simulink model "VDSE_2019a"  (R2019a)
settings: Solver=ode5  StartTime=0.0  StopTime=T_simulation  FixedStep=simulation_step_time  RelTol=1e-3
values from neighbouring files (symbols this model uses):
  A = 2    [vehicle_parameters_script.m]
  bump_height = 0    [vehicle_parameters_script.m]
  bump_length = 1    [vehicle_parameters_script.m]
  bump_time = 1    [vehicle_parameters_script.m]
  Bxf = 17.156    [BCD_Parameters.m]
  Bxr = 17.156    [BCD_Parameters.m]
  Byf = 12.71    [BCD_Parameters.m]
  Byr = 12.71    [BCD_Parameters.m]
  cd = 0.35    [vehicle_parameters_script.m]
  central_diff = 1    [vehicle_parameters_script.m]
  cF = 5000    [vehicle_parameters_script.m]
  clF = -0.15    [vehicle_parameters_script.m]
  clR = -0.20    (= -0.2)    [vehicle_parameters_script.m]
  cp_FA = 30    [vehicle_parameters_script.m]
  cp_RA = 13    [vehicle_parameters_script.m]
  cR = 5000    [vehicle_parameters_script.m]
  ctF = tireF.VERTICAL_DAMPING    [vehicle_parameters_script.m]
  ctR = tireR.VERTICAL_DAMPING    [vehicle_parameters_script.m]
  Cxf = 1.406    [BCD_Parameters.m]
  Cxr = 1.406    [BCD_Parameters.m]
  Cyf = 1.63    [BCD_Parameters.m]
  Cyr = 1.63    [BCD_Parameters.m]
  Dxf = 1.2    [BCD_Parameters.m]
  Dxr = 1.2    [BCD_Parameters.m]
  Dyf = 1.1    [BCD_Parameters.m]
  Dyr = 1.8    [BCD_Parameters.m]
  enableDriverControl = 0    [vehicle_parameters_script.m]
  enableLongDynamics = 1    [vehicle_parameters_script.m]
  enablePowertrain = 1    [vehicle_parameters_script.m]
  front_dr = 3.8    [vehicle_parameters_script.m]
  g = 9.806    [vehicle_parameters_script.m]
  Gear_numbers = [1 2 3 4 5 6]    [vehicle_parameters_script.m]
  GR = [2.9 1.8 1.3 1 0.85 0.75]    [vehicle_parameters_script.m]
  hcog = 0.5    [vehicle_parameters_script.m]
  hpc = 0.0    (= 0)    [vehicle_parameters_script.m]
  hrcF = 0.3    [vehicle_parameters_script.m]
  hrcg = (hrcF*lR+hrcR*lF)/(lF+lR)    (= 0.25108)    [vehicle_parameters_script.m]
  hrcR = 0.2    [vehicle_parameters_script.m]
  huFcog = 0.32    [vehicle_parameters_script.m]
  huRcog = 0.32    [vehicle_parameters_script.m]
  initial_gear = 1    [vehicle_parameters_script.m]
  JwF = 2.45    [vehicle_parameters_script.m]
  JwR = 2.45    [vehicle_parameters_script.m]
  Jx = 430    [vehicle_parameters_script.m]
  Jy = 1309    [vehicle_parameters_script.m]
  Jz = 1461    [vehicle_parameters_script.m]
  kF = 40000    [vehicle_parameters_script.m]
  kR = 35000    [vehicle_parameters_script.m]
  kRF = 0    [vehicle_parameters_script.m]
  kRR = 0    [vehicle_parameters_script.m]
  ktF = tireF.VERTICAL_STIFFNESS    [vehicle_parameters_script.m]
  ktR = tireR.VERTICAL_STIFFNESS    [vehicle_parameters_script.m]
  lF = 1.223    [vehicle_parameters_script.m]
  lR = l-lF    (= 1.277)    [vehicle_parameters_script.m]
  m = 1310    [vehicle_parameters_script.m]
  max_pressure = 1000    [vehicle_parameters_script.m]
  maxrpm = 4000    [vehicle_parameters_script.m]
  mF = 45    [vehicle_parameters_script.m]
  minrpm = 1500    [vehicle_parameters_script.m]
  mR = 50    [vehicle_parameters_script.m]
  output_samping_time = 0.001    [vehicle_parameters_script.m]
  phi0 = 0    [vehicle_parameters_script.m]
  phi_dot0 = 0    [vehicle_parameters_script.m]
  psi0 = 0    [vehicle_parameters_script.m]
  psi_dot0 = 0    [vehicle_parameters_script.m]
  rear_dr = 3.8    [vehicle_parameters_script.m]
  requested_speed = 100/3.6    (= 27.7777777778)    [vehicle_parameters_script.m]
  rF = tireF.UNLOADED_RADIUS    [vehicle_parameters_script.m]
  rho = 1.2    [vehicle_parameters_script.m]
  RPMME = Engine(:,1)    [vehicle_parameters_script.m]
  rR = tireR.UNLOADED_RADIUS    [vehicle_parameters_script.m]
  steer_ratio = 13.25    [vehicle_parameters_script.m]
  TFL = 0    [vehicle_parameters_script.m]
  TFR = 0    [vehicle_parameters_script.m]
  theta0 = 0    [vehicle_parameters_script.m]
  theta_dot0 = 0    [vehicle_parameters_script.m]
  TorqueME = []    [vehicle_parameters_script.m]
  TRL = 0    [vehicle_parameters_script.m]
  TRR = 0    [vehicle_parameters_script.m]
  Vx0 = 100/3.6    (= 27.7777777778)    [vehicle_parameters_script.m]
  Vy0 = 0    [vehicle_parameters_script.m]
  Vz0 = 0    [vehicle_parameters_script.m]
  wF = 1.578    [vehicle_parameters_script.m]
  wR = 1.544    [vehicle_parameters_script.m]
  x0 = 0    [vehicle_parameters_script.m]
  xcog_overall = (2*mR*xR+2*xF*mF+m*xs)/(m+2*mF+2*mR)    (= 1.23475333333)    [vehicle_parameters_script.m]
  y0 = 0    [vehicle_parameters_script.m]
  z0 = 0    [vehicle_parameters_script.m]
  zFL0 = 0    [vehicle_parameters_script.m]
  zFL_dot0 = 0    [vehicle_parameters_script.m]
  zFR0 = 0    [vehicle_parameters_script.m]
  zFR_dot0 = 0    [vehicle_parameters_script.m]
  zRL0 = 0    [vehicle_parameters_script.m]
  zRL_dot0 = 0    [vehicle_parameters_script.m]
  zRR0 = 0    [vehicle_parameters_script.m]
  zRR_dot0 = 0    [vehicle_parameters_script.m]
undefined symbols (not defined in the file or in its folder): exf, exr, eyf, eyr, FNOMINf, FNOMINr, PCX1f, PCX1r, PCY1f, PCY1r, PDX1f, PDX1r, PDX2f, PDX2r, PDY1f, PDY1r, PDY2f, PDY2r, PDY3f, PDY3r, PEX1f, PEX1r, PEX2f, PEX2r, PEX3f, PEX3r, PEX4f, PEX4r, PEY1f, PEY1r, PEY2f, PEY2r, PEY3f, PEY3r, PEY4f, PEY4r, PHX1f, PHX1r, PHX2f, PHX2r, PHY1f, PHY1r, PHY2f, PHY2r, PHY3f, PHY3r, PKX1f, PKX1r, PKX2f, PKX2r, PKX3f, PKX3r, PKY1f, PKY1r, PKY2f, PKY2r, PKY3f, PKY3r, PVX1f, PVX1r ... (+122)
libraries: simulink x7, mfeval_LIB x4
(part 5 of 6)

== matlab function VDSE_2019a/14-DOF VEHICLE MODEL/WHEEL ASSEMBLY/WHEEL ASSEMBLY MFEVAL/TIRE VELOCITIES ==
  data: deltaFL input; VFLx output; VFLy output; VFRx output; VFRy output; VRLx output; VRLy output; VRRx output; deltaFR input; deltaRL input; deltaRR input; V input; beta input; psidot input; VRRy output; lF input; lR input; wFL input; wFR input; wRL input; wRR input
function [VFLx, VFLy, VFRx, VFRy, VRLx, VRLy, VRRx, VRRy] = ConversiontoCorners(deltaFL,deltaFR,deltaRL,deltaRR,...
    V, beta, psidot,  lF, lR, wFL, wFR, wRL, wRR)
% Geometric calcs
lFL = sqrt(lF^2+wFL^2); gammaFL = atan2(wFL,lF);
lFR = sqrt(lF^2+wFR^2); gammaFR = atan2(wFR,lF);
lRL = sqrt(lR^2+wRL^2); gammaRL = atan2(wRL,lR);
lRR = sqrt(lR^2+wRR^2); gammaRR = atan2(wRR,lR);

VFLx = V*cos(deltaFL - beta) - psidot*lFL*sin(gammaFL - deltaFL);
VFLy = - V*sin(deltaFL - beta) + psidot*lFL*cos(gammaFL - deltaFL);
VFRx = V*cos(deltaFR - beta) + psidot*lFR*sin(gammaFR + deltaFR);
VFRy = - V*sin(deltaFR - beta) + psidot*lFR*cos(gammaFR + deltaFR);
VRLx = V*cos(deltaRL - beta) - psidot*lRL*sin(gammaRL + deltaRL);
VRLy = -V*sin(deltaRL - beta) - psidot*lRL*cos(gammaRL + deltaRL);
VRRx = V*cos(deltaRR - beta) + psidot*lRR*sin(gammaRR - deltaRR);
VRRy = -V*sin(deltaRR - beta) - psidot*lRR*cos(gammaRR - deltaRR);

end

== matlab function VDSE_2019a/14-DOF VEHICLE MODEL/WHEEL ASSEMBLY/WHEEL ASSEMBLY MFEVAL/WHEEL DYNAMICS ==
  data: rF input; rR input; JwF input; JwR input; omega_dot output size=[1 4]; fFLx input; fFRx input; fRLx input; fRRx input; TFL input; TFR input; TRL input; TRR input
function omega_dot  = TIRES(rF, rR, JwF, JwR, fFLx, fFRx, fRLx, fRRx,TFL,TFR,TRL,TRR)

%Wheel Dynamics
domegaFL = (TFL - fFLx*rF)/(JwF);
domegaFR = (TFR - fFRx*rF)/(JwF);
domegaRL = (TRL - fRLx*rR)/(JwR);
domegaRR = (TRR - fRRx*rR)/(JwR);

omega_dot = [domegaFL, domegaFR, domegaRL, domegaRR];

end

== matlab function VDSE_2019a/14-DOF VEHICLE MODEL/SUSPENSION/REAR SUSPENSION/SUSPENSION RL/RL/MATLAB Function ==
  data: mR input; wR input; lR input; cR input; kR input; kRR input; ctR input; ktR input; g input; yRL_road input; yRL_road_dot input; zRL_dot_dot output; z input; Vz input; phi input; phi_dot input; theta input; theta_dot input; zRR input; zRL input; zRL_dot input
function zRL_dot_dot = zRL(mR,wR,lR,cR,kR,kRR,ctR,ktR,g,yRL_road,yRL_road_dot,z,Vz,phi,phi_dot,theta,theta_dot,zRR,zRL,zRL_dot)
% Parameters:
% mR = half rear unsprung mass [kg]
% cR = rear damping damping rate [Ns/m]
% kR = rear spring stiffness [N/m]
% kRR = rear antiroll bar stiffness [N/m]
% wR = rear trackwidth [m]
% g = gravitational acceleration [m/s^2]
%
% Annotations:
% z = sprung mass vertical displacement [m]
% Vz = sprung mass vertical velocity [m/s]
% zij = unsprung vertical displacement [m]
% zij_dot = unsprung vertical velocity [m/s]
% zij_dot_dot = unsprung vertical acceleration [m/s^2]
% theta = pitch angle [rad]
% theta_dot = pitch angular velocity [rad/s]
% phi = roll angle [rad]
% phi_dot  = roll angular velocity [rad/s]
% y_rear_road = rear axle's road input displacement [m]
% y_rear_road_dot = rear axle's road input velocity [m/s]
%
% i: F, R = Front, Rear
% j: R, L = Right, Left

% Summation of forces:
sum = -cR*(Vz-zRL_dot+wR/2*phi_dot+lR*theta_dot) - kR*(z-zRL+wR/2*phi+lR*theta) - kRR/wR*(phi-(zRL-zRR)/wR) ...
    +ktR*(zRL-yRL_road)+ctR*(zRL_dot-yRL_road_dot)+mR*g;

% Calculation of RR unsprung mass vertical acceleration:
zRL_dot_dot = -sum/mR;

end

== matlab function VDSE_2019a/14-DOF VEHICLE MODEL/SUSPENSION/REAR SUSPENSION/SUSPENSION RR/RR/MATLAB Function ==
  data: mR input; wR input; lR input; cR input; kR input; kRR input; ctR input; ktR input; g input; yRR_road input; yRR_road_dot input; zRR_dot_dot output; z input; Vz input; phi input; phi_dot input; theta input; theta_dot input; zRL input; zRR input; zRR_dot input
function zRR_dot_dot = zRR(mR,wR,lR,cR,kR,kRR,ctR,ktR,g,yRR_road,yRR_road_dot,z,Vz,phi,phi_dot,theta,theta_dot,zRL,zRR,zRR_dot)
% Parameters:
% mR = half rear unsprung mass [kg]
% cR = rear damping damping rate [Ns/m]
% kR = rear spring stiffness [N/m]
% kRR = rear antiroll bar stiffness [N/m]
% wR = rear trackwidth [m]
% g = gravitational acceleration [m/s^2]
%
% Annotations:
% z = sprung mass vertical displacement [m]
% Vz = sprung mass vertical velocity [m/s]
% zij = unsprung vertical displacement [m]
% zij_dot = unsprung vertical velocity [m/s]
% zij_dot_dot = unsprung vertical acceleration [m/s^2]
% theta = pitch angle [rad]
% theta_dot = pitch angular velocity [rad/s]
% phi = roll angle [rad]
% phi_dot  = roll angular velocity [rad/s]
% y_rear_road = rear axle's road input displacement [m]
% y_rear_road_dot = rear axle's road input velocity [m/s]
%
% i: F, R = Front, Rear
% j: R, L = Right, Left

% Summation of forces:
sum = -cR*(Vz-zRR_dot-wR/2*phi_dot+lR*theta_dot) - kR*(z-zRR-wR/2*phi+lR*theta)...
    +kRR/wR*(phi - (zRL-zRR)/wR)+ktR*(zRR-yRR_road)+ ctR*(zRR_dot-yRR_road_dot) + mR*g;
% Calculation of RR unsprung mass vertical acceleration:
zRR_dot_dot = -sum/mR; 

end

== matlab function VDSE_2019a/14-DOF VEHICLE MODEL/EQUATIONS OF MOTION FOR CHASSIS/Vertical Dynamics/VERTICAL DYNAMICS ==
  data: m input; g input; lF input; Vz_dot output; lR input; wF input; wR input; kF input; kR input; cF input; cR input; phi input; phi_dot input; theta input; theta_dot input; zFL input; zFL_dot input; zFR input; zFR_dot input; zRL input; zRL_dot input; zRR input; zRR_dot input; Vx input; Vy input; fFLz_aero input; fFRz_aero input; fRLz_aero input; fRRz_aero input; z input; z_dot input
function Vz_dot = vertical_dynamics(m,g,lF,lR,wF,wR,kF,kR,cF,cR,phi,phi_dot,...
    theta,theta_dot,zFL,zFL_dot,zFR,zFR_dot,zRL,zRL_dot,zRR,zRR_dot,Vx,Vy,...
    fFLz_aero, fFRz_aero, fRLz_aero, fRRz_aero,z,z_dot)
% Parameters:
% m = sprung mass [kg]
% cF = front damping damping rate [Ns/m]
% cR = rear damping damping rate [Ns/m]
% kF = front spring stiffness [N/m]
% kR = rear spring stiffness [N/m]
% lF = front wheel base [m]
% lR = rear wheel base [m]
% wF = front trackwidth [m]
% wR = rear trackwidth [m]
% g = gravitational acceleration [m/s^2]
%
% Annotations:
% z = sprung mass vertical displacement [m]
% Vz = sprung mass vertical velocity [m/s]
% Vz_dot = sprung mass vertical acceleration [m/s^2]
% zij = unsprung vertical displacement [m]
% zij_dot = unsprung vertical velocity [m/s]
% fijz_aero = downforces applied on the chassis [N]
% theta = pitch angle [rad]
% theta_dot = pitch angular velocity [rad/s]
% phi = roll angle [rad]
% phi_dot  = roll angular velocity [rad/s]
% Vy = vehicle's lateral velocity [m/s]
% Vx = vehicle's longitudinal velocity [m/s]
%
% i: F, R = Front, Rear
% j: R, L = Right, Left

% Summation of forces:
sum=cF*(z_dot-zFL_dot+(wF/2)*phi_dot-lF*theta_dot)...
    +cF*(z_dot-zFR_dot-(wF/2)*phi_dot-lF*theta_dot)...
    +cR*(z_dot-zRL_dot+(wR/2)*phi_dot+lR*theta_dot)...
    +cR*(z_dot-zRR_dot-(wR/2)*phi_dot+lR*theta_dot)...
    +kF*(z-zFL+(wF/2)*phi-lF*theta)...
    +kF*(z-zFR-(wF/2)*phi-lF*theta)...
    +kR*(z-zRL+(wR/2)*phi+lR*theta)...
    +kR*(z-zRR-(wR/2)*phi+lR*theta)...
    +m*g+m*Vx*theta_dot-m*Vy*phi_dot...
    +fFLz_aero+fFRz_aero+fRLz_aero+fRRz_aero;

% Calculation of vertical acceleration of sprung mass (including tangential terms):
Vz_dot=-sum/m;
end

== matlab function VDSE_2019a/14-DOF VEHICLE MODEL/EQUATIONS OF MOTION FOR CHASSIS/Roll Dynamics/ROLL DYNAMICS ==
  data: Jx input; g input; lF input; phi_dot_dot output; lR input; wF input; wR input; kF input; kR input; kRF input; kRR input; cF input; cR input; z input; z_dot input; theta input; theta_dot input; zFL input; zFL_dot input; zFR input; zFR_dot input; zRL input; zRL_dot input; zRR input; zRR_dot input; ay input; hrcg input; hcog input; m input; fFLz_aero input; fFRz_aero input; fRLz_aero input; fRRz_aero input; phi input; phi_dot input
function phi_dot_dot = roll_dynamics(Jx,g,lF,lR,wF,wR,kF,kR,kRF,kRR,cF,cR,z,z_dot,theta,theta_dot,...
    zFL,zFL_dot,zFR,zFR_dot,zRL,zRL_dot,zRR,zRR_dot,ay,hrcg,hcog,m,...
    fFLz_aero,fFRz_aero,fRLz_aero,fRRz_aero,phi,phi_dot)

% Parameters:
% m = sprung mass [kg]
% Jx = roll moment of inertial [kgm^2]
% cF = front damping damping rate [Ns/m]
% cR = rear damping damping rate [Ns/m]
% kF = front spring stiffness [N/m]
% kR = rear spring stiffness [N/m]
% kRF = front antiroll bar stiffness [N/m]
% kRR = front antiroll bar stiffness [N/m]
% lF = front wheel base [m]
% lR = rear wheel base [m]
% wF = front trackwidth [m]
% wR = rear trackwidth [m]
% hrcg = roll center height at the center of gravity [m]
% hcog = height of center of gravity [m]
% g = gravitational acceleration [m/s^2]
%
% Annotations:
% z = sprung mass vertical displacement [m]
% Vz = sprung mass vertical velocity [m/s]
% Vz_dot = sprung mass vertical acceleration [m/s^2]
% zij = unsprung vertical displacement [m]
% zij_dot = unsprung vertical velocity [m/s]
% fijz_aero = downforces applied on the chassis [N]
% theta = pitch angle [rad]
% theta_dot = pitch angular velocity [rad/s]
% phi = roll angle [rad]
% phi_dot  = roll angular velocity [rad/s]
% ay = vehicle's overall lateral acceleration [m/s^2]
%
% i: F, R = Front, Rear
% j: R, L = Right, Left

% Summation of moments:
sumF=(wF/2)*cF*(z_dot-zFL_dot+(wF/2)*phi_dot-lF*theta_dot)...
    -(wF/2)*cF*(z_dot-zFR_dot-(wF/2)*phi_dot-lF*theta_dot)...
    +(wR/2)*cR*(z_dot-zRL_dot+(wR/2)*phi_dot+lR*theta_dot)...
    -(wR/2)*cR*(z_dot-zRR_dot-(wR/2)*phi_dot+lR*theta_dot)...
    +(wF/2)*kF*(z-zFL+(wF/2)*phi-lF*theta)...
    -(wF/2)*kF*(z-zFR-(wF/2)*phi-lF*theta)...
    +(wR/2)*kR*(z-zRL+(wR/2)*phi+lR*theta)...
    -(wR/2)*kR*(z-zRR-(wR/2)*phi+lR*theta)...
    +kRF*(phi-(zFL-zFR)/wF)...
    +kRR*(phi-(zRL-zRR)/wR)-m*(hcog-hrcg)*ay*cos(phi)-m*g*(hcog-hrcg)*sin(phi)...
    -wF*fFLz_aero+wF*fFRz_aero-wR*fRLz_aero+wR*fRRz_aero;

% Roll angular acceleration calculation:
phi_dot_dot=-sumF/(Jx+m*(hcog-hrcg)^2);
end

== matlab function VDSE_2019a/14-DOF VEHICLE MODEL/EQUATIONS OF MOTION FOR CHASSIS/Pitch Dynamics/PITCH DYNAMICS ==
  data: Jy input; g input; lF input; theta_dot_dot output; lR input; wF input; wR input; kF input; kR input; cF input; cR input; z input; z_dot input; phi input; phi_dot input; zFL input; zFL_dot input; zFR input; zFR_dot input; zRL input; zRL_dot input; zRR input; zRR_dot input; ax input; hpc input; hcog input; m input; fFLz_aero input; fFRz_aero input; fRLz_aero input; fRRz_aero input; theta input; theta_dot input
function theta_dot_dot = pitch_dynamics(Jy,g,lF,lR,wF,wR,kF,kR,cF,cR,z,z_dot,phi,phi_dot,...
    zFL,zFL_dot,zFR,zFR_dot,zRL,zRL_dot,zRR,zRR_dot,ax,hpc,hcog,m,...
    fFLz_aero,fFRz_aero,fRLz_aero,fRRz_aero,theta, theta_dot)
% Parameters:
% m = sprung mass [kg]
% Jy = pitch moment of inertial [kgm^2]
% cF = front damping damping rate [Ns/m]
% cR = rear damping damping rate [Ns/m]
% kF = front spring stiffness [N/m]
% kR = rear spring stiffness [N/m]
% lF = front wheel base [m]
% lR = rear wheel base [m]
% wF = front trackwidth [m]
% wR = rear trackwidth [m]
% hpc = pitch center height at the center of gravity [m]
% hcog = height of center of gravity [m]
% g = gravitational acceleration [m/s^2]
%
% Annotations:
% z = sprung mass vertical displacement [m]
% Vz = sprung mass vertical velocity [m/s]
% Vz_dot = sprung mass vertical acceleration [m/s^2]
% zij = unsprung vertical displacement [m]
% zij_dot = unsprung vertical velocity [m/s]
% fijz_aero = downforces applied on the chassis [N]
% theta = pitch angle [rad]
% theta_dot = pitch angular velocity [rad/s]
% phi = roll angle [rad]
% phi_dot  = roll angular velocity [rad/s]
% ax = vehicle's overall longitudinal acceleration [m/s^2]
%
% i: F, R = Front, Rear
% j: R, L = Right, Left

% Summation of moments:
sumF=-lF*cF*(z_dot-zFL_dot+(wF/2)*phi_dot-lF*theta_dot)...
    -lF*cF*(z_dot-zFR_dot-(wF/2)*phi_dot-lF*theta_dot)...
    +lR*cR*(z_dot-zRL_dot+(wR/2)*phi_dot+lR*theta_dot)...
    +lR*cR*(z_dot-zRR_dot-(wR/2)*phi_dot+lR*theta_dot)...
    -lF*kF*(z-zFL+(wF/2)*phi-lF*theta)...
    -lF*kF*(z-zFR-(wF/2)*phi-lF*theta)...
    +lR*kR*(z-zRL+(wR/2)*phi+lR*theta)...
    +lR*kR*(z-zRR-(wR/2)*phi+lR*theta)-m*(hcog-hpc)*ax*cos(theta)-m*g*(hcog-hpc)*sin(theta)...
    -lF*fFLz_aero-lF*fFRz_aero+lR*fRLz_aero+lR*fRRz_aero;
      
theta_dot_dot=-sumF/(Jy+m*(hcog-hpc)^2);
end

== matlab function VDSE_2019a/14-DOF VEHICLE MODEL/WHEEL ASSEMBLY/WHEEL ASSEMBLY BCD/TIRE FORCES AND WHEEL DYNAMICS ==
  data: rF input; rR input; JwF input; JwR input; fFLz input; fFRz input; fRLz input; fRRz input; omegaFL input; omegaFR input; omegaRL input; omegaRR input; fFLx output; fFRx output; fRLx output; fRRx output; VFLx input; VFLy input; VFRx input; VFRy input; VRLx input; VRLy input; VRRx input; VRRy input; fFLy output; fFRy output; fRLy output; fRRy output; omega_dot output size=[1 4]; TFL input; TFR input; TRL input; TRR input; TireParams input
function [fFLx, fFRx, fRLx,fRRx, fFLy,  fFRy, fRLy, fRRy, omega_dot] = TIRES(rF, rR, JwF, JwR,...
    fFLz, fFRz, fRLz, fRRz,...
    omegaFL, omegaFR, omegaRL, omegaRR, ...
    VFLx, VFLy, VFRx, VFRy, VRLx, VRLy, VRRx, VRRy, TFL, TFR, TRL, TRR, TireParams)
% Longitudinal slip:
sFLx = (VFLx - omegaFL*rF)/abs(omegaFL*rF);
sFRx = (VFRx - omegaFR*rF)/abs(omegaFR*rF);
sRLx = (VRLx - omegaRL*rR)/abs(omegaRL*rR);
sRRx = (VRRx - omegaRR*rR)/abs(omegaRR*rR);


% Lateral slip:
if VFLx==0
    sFLy = 0;
else
    sFLy = (1 + sFLx)*VFLy/abs(VFLx);
end

if VFRx==0
    sFRy = 0;
else
    sFRy = (1 + sFRx)*VFRy/abs(VFRx);
end

if VRLx==0
    sRLy = 0;
else
    sRLy = (1 + sRLx)*VRLy/abs(VRLx);
end

if VRRx == 0
    sRRy = 0;
else
 
    sRRy = (1 + sRRx)*VRRy/abs(VRRx);
end

% Total slip:
sFL = sqrt(sFLx^2 + sFLy^2);
sFR = sqrt(sFRx^2 + sFRy^2);
sRL = sqrt(sRLx^2 + sRLy^2);
sRR = sqrt(sRRx^2 + sRRy^2);

%Tire parameters
Bxf = TireParams(1);
Cxf = TireParams(2);
Dxf = TireParams(3);
Bxr = TireParams(4);
Cxr = TireParams(5);
Dxr = TireParams(6);
Byf = TireParams(7);
Cyf = TireParams(8);
Dyf = TireParams(9);
Byr = TireParams(10);
Cyr = TireParams(11);
Dyr = TireParams(12);

% BCD Version - Longitudinal:
muFLx = Dxf*sin(Cxf*atan(Bxf*sFL));
muFRx = Dxf*sin(Cxf*atan(Bxf*sFR));
muRLx = Dxr*sin(Cxr*atan(Bxr*sRL));
muRRx = Dxr*sin(Cxr*atan(Bxr*sRR));


% % BCD Version - Lateral:
muFLy = Dyf*sin(Cyf*atan(Byf*sFL));
muFRy = Dyf*sin(Cyf*atan(Byf*sFR));
muRLy = Dyr*sin(Cyr*atan(Byr*sRL));
muRRy = Dyr*sin(Cyr*atan(Byr*sRR));


if sFL == 0
muFLx_long = 0;
muFLy_lat = 0;
else
muFLx_long = -sFLx*muFLx/sFL;
muFLy_lat = -sFLy*muFLy/sFL;
end

if sFR == 0
muFRx_long = 0;
muFRy_lat = 0;
else
muFRx_long = -sFRx*muFRx/sFR;
muFRy_lat = -sFRy*muFRy/sFR;
end

if sRL == 0
muRLx_long = 0;
muRLy_lat = 0;
else
muRLx_long = -sRLx*muRLx/sRL;
muRLy_lat = -sRLy*muRLy/sRL;
end

if sRR == 0
muRRx_long = 0;
muRRy_lat = 0;
else    
muRRx_long = -sRRx*muRRx/sRR;
muRRy_lat = -sRRy*muRRy/sRR;
end

fFLx = fFLz*muFLx_long; fFLy = fFLz*muFLy_lat;
fFRx = fFRz*muFRx_long; fFRy = fFRz*muFRy_lat;
fRLx = fRLz*muRLx_long; fRLy = fRLz*muRLy_lat;
fRRx = fRRz*muRRx_long; fRRy = fRRz*muRRy_lat;

%Wheel Dynamics
domegaFL = (TFL - fFLx*rF)/(JwF);
domegaFR = (TFR - fFRx*rF)/(JwF);
domegaRL = (TRL - fRLx*rR)/(JwR);
domegaRR = (TRR - fRRx*rR)/(JwR);

omega_dot = [domegaFL, domegaFR, domegaRL, domegaRR];

end

== matlab function VDSE_2019a/14-DOF VEHICLE MODEL/WHEEL ASSEMBLY/WHEEL ASSEMBLY BCD/TIRE VELOCITIES ==
  data: deltaFL input; VFLx output; VFLy output; VFRx output; VFRy output; VRLx output; VRLy output; VRRx output; deltaFR input; deltaRL input; deltaRR input; V input; beta input; psidot input; lF input; lR input; VRRy output; wFL input; wFR input; wRL input; wRR input
function [VFLx, VFLy, VFRx, VFRy, VRLx, VRLy, VRRx, VRRy] = ConversiontoCorners(deltaFL,deltaFR,deltaRL,deltaRR,...
    V, beta, psidot,  lF, lR, wFL, wFR, wRL, wRR)
% Geometric calcs
lFL = sqrt(lF^2+wFL^2); gammaFL = atan2(wFL,lF);
lFR = sqrt(lF^2+wFR^2); gammaFR = atan2(wFR,lF);
lRL = sqrt(lR^2+wRL^2); gammaRL = atan2(wRL,lR);
lRR = sqrt(lR^2+wRR^2); gammaRR = atan2(wRR,lR);

% Tire Velocities
VFLx = V*cos(deltaFL - beta) - psidot*lFL*sin(gammaFL - deltaFL);
VFLy = - V*sin(deltaFL - beta) + psidot*lFL*cos(gammaFL - deltaFL);
VFRx = V*cos(deltaFR - beta) + psidot*lFR*sin(gammaFR + deltaFR);
VFRy = - V*sin(deltaFR - beta) + psidot*lFR*cos(gammaFR + deltaFR);
VRLx = V*cos(deltaRL - beta) - psidot*lRL*sin(gammaRL + deltaRL);
VRLy = -V*sin(deltaRL - beta) - psidot*lRL*cos(gammaRL + deltaRL);
VRRx = V*cos(deltaRR - beta) + psidot*lRR*sin(gammaRR - deltaRR);
VRRy = -V*sin(deltaRR - beta) - psidot*lRR*cos(gammaRR - deltaRR);
end

== matlab function VDSE_2019a/14-DOF VEHICLE MODEL/EQUATIONS OF MOTION FOR CHASSIS/Longitudinal Dynamics/LONGIDUTINAL DYNAMICS ==
  data: deltaFL input; ax output; fFLx input; fFLy input; deltaFR input; fFRx input; fFRy input; deltaRL input; fRLx input; fRLy input; deltaRR input; fRRx input; fRRy input; mFLy input; mFRy input; mRLy input; mRRy input; Vy input; psi_dot input; theta_dot input; Vz input; Vx input; m input; mF input; mR input; rho input; cd input; A input; rF input; rR input; Vx_dot output
function [ax, Vx_dot] = longitudinal_dynamics(deltaFL, fFLx, fFLy, deltaFR, fFRx, fFRy, deltaRL, fRLx, fRLy, deltaRR, fRRx, fRRy,mFLy,mFRy,mRLy,mRRy, ...
    Vy, psi_dot, theta_dot, Vz, Vx, m, mF, mR,rho,cd,A,rF,rR)

% Parameters:
% m = sprung mass [kg]
% mF = half front unsprung mass [kg]
% mR = half rear unsprung mass [kg]
% rho = air density [kg/m^3]
% cd = drag coefficient [-]
% A = vehicle's frontal area [m^2]
% rF = front dynamic radius [m]
% rR = rear dynamic radius [m]
%
% Annotations:
% fijx, fijy = force at the tire frame [N]
% mijy = rolling moment at the tire frame [Nm]
% ax = overall longidutinal acceleration [m/s^2]
% Vx_dot = longidutinal acceleration excluding tangential terms [m/s^2]
% theta_dot = pitch angular velocity [rad/s]
% psi_dot = yaw angular velocity [rad/s]
% Vz = vertical sprung mass velocity [m/s]
% Vy = lateral vehicle's velocity [m/s]
% Vx = longitudinal vehicle's velocity [m/s]
% deltaFL = FL wheel's steering angle [rad]
% deltaFR = FR wheel's steering angle [rad]
% deltaRL = RL wheel's steering angle [rad]
% deltaRR = RR wheel's steering angle [rad]
%
% i: F, R = Front, Rear
% j: R, L = Right, Left

% Projection in the vehicle frame:
fFLx_vehicle=fFLx*cos(deltaFL)-fFLy*sin(deltaFL);  
fFRx_vehicle=fFRx*cos(deltaFR)-fFRy*sin(deltaFR);
fRLx_vehicle=fRLx*cos(deltaRL)-fRLy*sin(deltaRL);
fRRx_vehicle=fRRx*cos(deltaRR)-fRRy*sin(deltaRR);

% Calculation of overall longitudinal acceleration:
ax = (fFLx_vehicle+fFRx_vehicle+fRLx_vehicle+fRRx_vehicle+mFLy/rF*cos(deltaFL)+mFRy/rF*cos(deltaFR)+...
    mRLy/rR*cos(deltaRL)+mRRy/rR*cos(deltaRR)-1/2*rho*cd*A*Vx^2)/(m+2*mR+2*mF);

% Calculation of vehicle's longitudinal acceleration excluding tangential terms: 
Vx_dot = ax - theta_dot*Vz + Vy*psi_dot;

end
